simulink model "Passive_Hydraulic_PTO_Sim"  (R2014a)
settings: Solver=ode23tb  StartTime=0.0  StopTime=param.stop  MaxStep=0.05  RelTol=1e-6
libraries: PTOSim_Lib x5
settings Model: Creator=sor  LastModifiedBy=sor

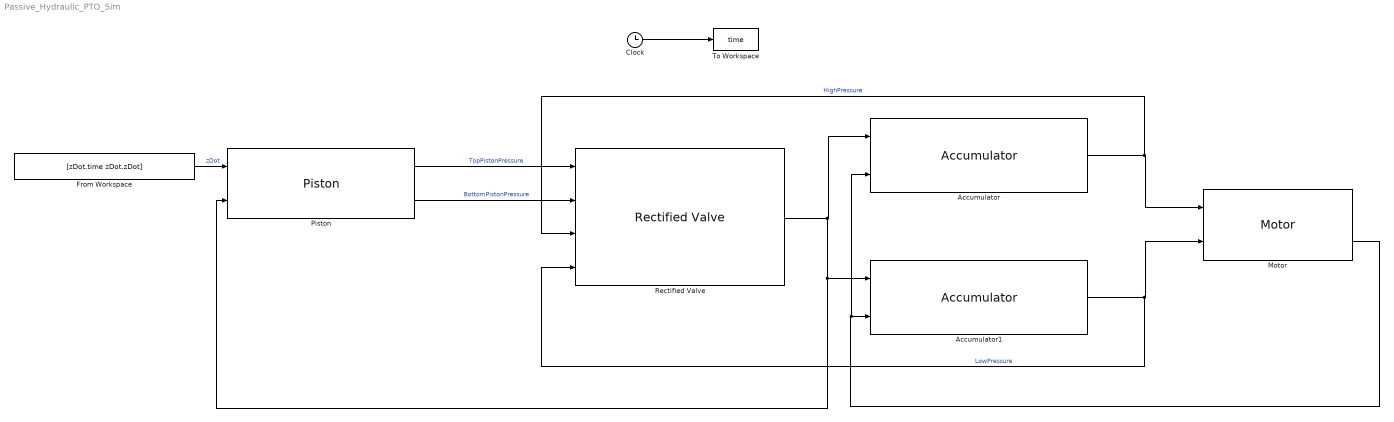
== system Passive_Hydraulic_PTO_Sim ==
  Accumulator : PTOSim_Lib/Hydraulic_PTO/Accumulator  OverrideUsingVariant=Variant  Parameter1=0
  Accumulator1 : PTOSim_Lib/Hydraulic_PTO/Accumulator  OverrideUsingVariant=Variant1  Parameter1=0
  Clock : Clock
  From Workspace : FromWorkspace  VariableName=[zDot.time zDot.zDot]  SampleTime=0  OutputAfterFinalValue=Holding final value
  "Motor " : PTOSim_Lib/Hydraulic_PTO/Motor   Parameter1=0
  "Piston " : PTOSim_Lib/Hydraulic_PTO/Piston    Parameter1=0
  Rectified Valve : PTOSim_Lib/Hydraulic_PTO/Rectified Valve  Parameter1=0
  To Workspace : ToWorkspace  VariableName=time  SampleTime=-1
  wires:
  "Piston "/1 -> Rectified Valve/1  "TopPistonPressure"
  "Piston "/2 -> Rectified Valve/2  "BottomPistonPressure"
  Rectified Valve/1 -> "Piston "/2, Accumulator1/1, Accumulator/1
  Accumulator/1 -> Rectified Valve/3, "Motor "/1  "HighPressure"
  Accumulator1/1 -> Rectified Valve/4, "Motor "/2  "LowPressure"
  "Motor "/2 -> Accumulator/2, Accumulator1/2
  From Workspace/1 -> "Piston "/1  "zDot"
  Clock/1 -> To Workspace/1
